simulink model "Dampler_System_with_PID"  (R2025b)
settings: Solver=VariableStepAuto  StartTime=0.0  StopTime=10.0  MaxStep=0.01  RelTol=1e-3
undefined symbols (not defined in the file or in its folder): b, k, Kd, Ki, Kp, M
settings Model: Creator=night  LastModifiedBy=night

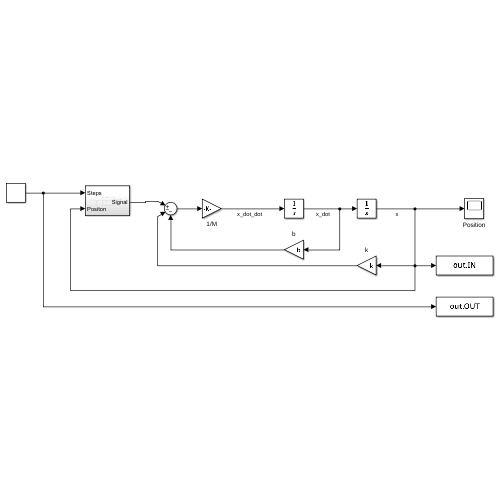
[thumbnail: Simulink's stored preview of the top-level diagram]
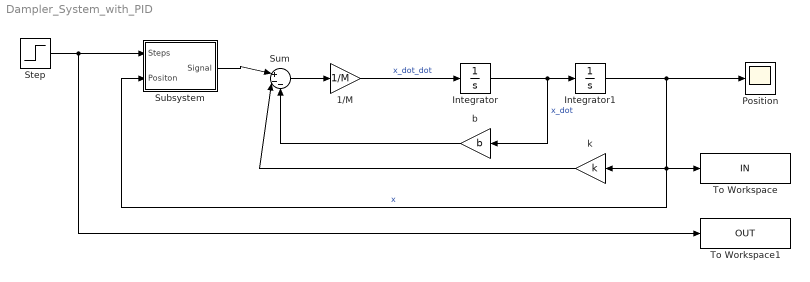
== system Dampler_System_with_PID ==
  1/M : Gain  Gain=1/M
  Integrator : Integrator
  Integrator1 : Integrator
  Position : Scope
      settings: ActiveDisplayYMinimum=-2.4661743957715032E+35  ActiveDisplayYMaximum=2.2195569561943532E+36
  Step : Step  SampleTime=0
  Subsystem : Subsystem
  Sum : Sum  Inputs=|+--
  To Workspace : ToWorkspace  VariableName=IN  SaveFormat=Timeseries  SampleTime=-1
  To Workspace1 : ToWorkspace  VariableName=OUT  SaveFormat=Timeseries  SampleTime=-1
  b : Gain  Gain=b
  k : Gain  Gain=k
  wires:
  Integrator/1 -> b/1, Integrator1/1  "x_dot"
  Subsystem/1(Signal) -> Sum/1
  k/1 -> Sum/2
  Integrator1/1 -> To Workspace/1, Subsystem/2(Positon), k/1, Position/1  "x"
  b/1 -> Sum/3
  1/M/1 -> Integrator/1  "x_dot_dot"
  Sum/1 -> 1/M/1
  Step/1 -> To Workspace1/1, Subsystem/1(Steps)

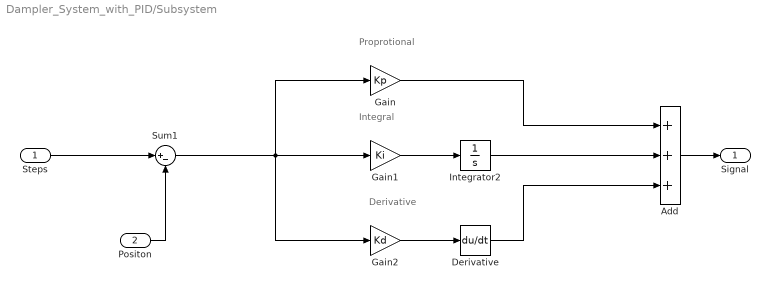
== system Dampler_System_with_PID/Subsystem ==
  note: Proprotional
  note: Integral
  note: Derivative
  Steps : Inport
  Positon : Inport  Port=2
  Add : Sum  Inputs=+++
  Derivative : Derivative
  Gain : Gain  Gain=Kp
  Gain1 : Gain  Gain=Ki
  Gain2 : Gain  Gain=Kd
  Integrator2 : Integrator
  Sum1 : Sum  Inputs=|+-
  Signal : Outport
  wires:
  Gain/1 -> Add/1
  Gain1/1 -> Integrator2/1
  Derivative/1 -> Add/3
  Gain2/1 -> Derivative/1
  Steps/1 -> Sum1/1
  Positon/1 -> Sum1/2
  Sum1/1 -> Gain2/1, Gain1/1, Gain/1
  Integrator2/1 -> Add/2
  Add/1 -> Signal/1
